simulink model "modelo_f_nico_local"  (R2024b)
settings: Solver=VariableStepAuto  StartTime=0.0  StopTime=100  RelTol=1e-3
InitFcn:
  | parametros
  | gain_CL
values from neighbouring files (symbols this model uses):
  Ah = [0 1 ... (first row only)    [calculo_observador_izaje.m]
  At = [ 0, 1, 0, 0 ... (first row only)    [calculo_observador_carro.m]
  b_cy = 1e7    (= 10000000)    [parametros.m]
  b_ha = -(J_hEq + (r_hd/(2*i_h))*m_l) * w_des_h*(1 + n_h + n_h^2) + b_hEq    [gain_CL.m]
  b_hb = 1e8    (= 100000000)    [parametros.m]
  b_hd = 8    [parametros.m]
  b_hEb = 2.2e9    (= 2200000000)    [parametros.m]
  b_hm = 18    [parametros.m]
  b_t = 90    [parametros.m]
  b_ta = M_tEq*w_des_t*(1+n_t+n_t^2)-b_tEq    [gain_CL.m]
  b_tb = 5e6    (= 5000000)    [parametros.m]
  b_td = 1.8    [parametros.m]
  b_tm = 6    [parametros.m]
  b_tw = 3e3    (= 3000)    [parametros.m]
  b_wu = 150    [parametros.m]
  Bch = [0 ... (first row only)    [calculo_observador_izaje.m]
  Bct = [ 0, 0 ... (first row only)    [calculo_observador_carro.m]
  Bdh = [0 ... (first row only)    [calculo_observador_izaje.m]
  Bdt = [ 0 ... (first row only)    [calculo_observador_carro.m]
  Ch = [1 0]    [calculo_observador_izaje.m]
  Ct = [ 1, 0, 0, 0 ]    [calculo_observador_carro.m]
  g = 9.80665    [parametros.m]
  i_h = 22    [parametros.m]
  i_t = 30    [parametros.m]
  J_hd_hEb = 3800    [parametros.m]
  J_hm_hb = 30    [parametros.m]
  J_td = 1200    [parametros.m]
  J_tm_tb = 7    [parametros.m]
  K_cy = 1.8e9    (= 1800000000)    [parametros.m]
  k_hsa = -(J_hEq + (r_hd/(2*i_h))*m_l) * w_des_h^2*(n_h + n_h^2 + n_h^3)    [gain_CL.m]
  k_hsia = -(J_hEq + (r_hd/(2*i_h))*m_l) * n_h^3 * w_des_h^3    [gain_CL.m]
  k_tsa = M_tEq*w_des_t^2*n_t*(1+n_t+n_t^2)    [gain_CL.m]
  k_tsia = M_tEq*w_des_t^3*n_t^3    [gain_CL.m]
  K_tw = 4.8e5    (= 480000)    [parametros.m]
  k_wu = 2.36e8    (= 236000000)    [parametros.m]
  l_h0 = (Y_t0-y_l0)    (= 5)    [parametros.m]
  Lh = place(Ah', Ch', polos_h)'    [calculo_observador_izaje.m]
  Lt = place(At', Ct', polos_deseados)'    [calculo_observador_carro.m]
  m_l = M_s+M_cmax    (= 65000)    [parametros.m]
  M_t = 30000    [parametros.m]
  M_tEq = i_t/r_td*(J_tm_tb+J_td/i_t^2)+r_td/i_t*(M_t+m_l)    (= 2083.33333333)    [parametros.m]
  r_hd = 0.75    [parametros.m]
  r_td = 0.50    (= 0.5)    [parametros.m]
  T_hbMax = 5e4    (= 50000)    [parametros.m]
  T_hEbMax = 1.1e6    (= 1100000)    [parametros.m]
  T_hmMax = 2e4    (= 20000)    [parametros.m]
  T_s = min([T_hs,T_ts])    [parametros.m]
  T_tbMax = 5e3    (= 5000)    [parametros.m]
  T_tmMax = 4e3    (= 4000)    [parametros.m]
  tau_tm = 1e-3    (= 0.001)    [parametros.m]
  theta_hm0 = -l_h0*i_h*2/r_hd    (= -293.333333333)    [parametros.m]
  theta_tm0 = (x_t0)*i_t/r_td    (= -1200)    [parametros.m]
  v_lx0 = 0    [parametros.m]
  v_ly0 = 0    [parametros.m]
  v_t0 = 0    [parametros.m]
  w_hm0 = 0    [parametros.m]
  w_hm_rated = v_h_max_load*2*i_h/r_hd    (= 88)    [parametros.m]
  w_tm0 = (v_t0)*i_t/r_td    (= 0)    [parametros.m]
  x_l0 = x_t0    (= -20)    [parametros.m]
  x_t0 = -20    [parametros.m]
  y_l0 = 40    [parametros.m]
  Y_t0 = 45    [parametros.m]
libraries: simulink x1
settings Model: Creator=nsorr  LastModifiedBy=nsorr

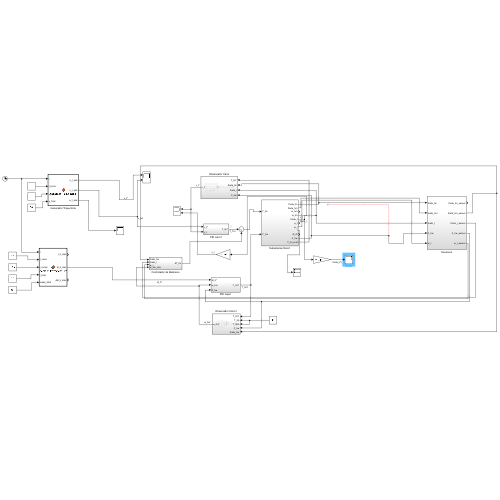
[thumbnail: Simulink's stored preview of the top-level diagram]
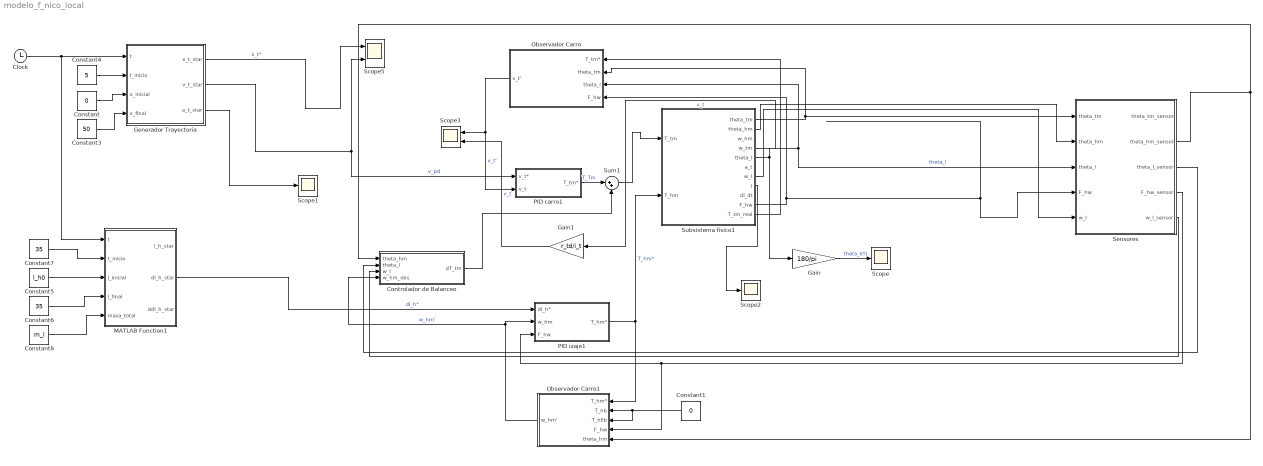
== system modelo_f_nico_local ==
  Clock : Clock
  Constant : Constant  Value=0
  Constant1 : Constant  Value=0
  Constant3 : Constant  Value=50
  Constant4 : Constant  Value=5
  Constant5 : Constant  Value=l_h0
  Constant6 : Constant  Value=35
  Constant7 : Constant  Value=35
  Constant8 : Constant  Value=m_l
  Controlador de Balanceo : Subsystem
  Gain : Gain  Gain=180/pi
  Gain1 : Gain  Gain=r_td/i_t
  Generador Trayectoria : MATLAB Function  TreatAsAtomicUnit=on
  MATLAB Function1 : MATLAB Function  TreatAsAtomicUnit=on
  Observador Carro : Subsystem
  Observador Carro1 : Subsystem
  PID carro1 : Subsystem
  PID izaje1 : Subsystem
  Scope : Scope
  Scope1 : Scope
  Scope2 : Scope
  Scope3 : Scope  NumInputPorts=2
  Scope5 : Scope  NumInputPorts=2
  Sensores : Subsystem
  Subsistema físico1 : Subsystem
  Sum1 : Sum  Inputs=|++
  wires:
  Generador Trayectoria/1(x_t_star) -> Scope5/1  "x_t*"
  MATLAB Function1/2(dl_h_star) -> PID izaje1/1(dl_h*)  "dl_h*"
  Subsistema físico1/2(theta_hm) -> Sensores/2(theta_hm)
  PID carro1/1(T_tm*) -> Sum1/1  "T_Tm"
  Subsistema físico1/8(l) -> Scope2/1
  Subsistema físico1/4(w_tm) -> Gain1/1  "v_t"
  Subsistema físico1/5(theta_l) -> Observador Carro/3(theta_l), Sensores/3(theta_l), Gain/1  "theta_l"
  PID izaje1/1(T_hm*) -> Observador Carro1/1(T_hm*), Subsistema físico1/2(T_hm)  "T_hm*"
  Gain/1 -> Scope/1  "theta_l(º)"
  Clock/1 -> MATLAB Function1/1(t), Generador Trayectoria/1(t)
  Constant/1 -> Generador Trayectoria/3(x_inicial)
  Constant3/1 -> Generador Trayectoria/4(x_final)
  Constant4/1 -> Generador Trayectoria/2(t_inicio)
  Constant5/1 -> MATLAB Function1/3(l_inicial)
  Constant6/1 -> MATLAB Function1/4(l_final)
  Constant7/1 -> MATLAB Function1/2(t_inicio)
  Constant8/1 -> MATLAB Function1/5(masa_total)
  Generador Trayectoria/2(v_t_star) -> PID carro1/1(v_t*), Scope5/2  "v_pd"
  Controlador de Balanceo/1(dT_tm) -> Sum1/2
  Sum1/1 -> Subsistema físico1/1(T_tm)
  Generador Trayectoria/3(a_t_star) -> Scope1/1
  Subsistema físico1/1(theta_tm) -> Observador Carro/2(theta_tm), Sensores/1(theta_tm)
  Subsistema físico1/10(F_hw) -> Observador Carro/4(F_hw), Sensores/4(F_hw)
  Subsistema físico1/7(w_l) -> Sensores/5(w_l)
  Sensores/5(w_l_sensor) -> Controlador de Balanceo/3(w_l)
  Sensores/3(theta_l_sensor) -> Controlador de Balanceo/2(theta_l)
  Sensores/2(theta_hm_sensor) -> Controlador de Balanceo/1(theta_hm), Observador Carro1/5(theta_hm)
  Sensores/4(F_hw_sensor) -> Observador Carro1/4(F_hw), PID izaje1/3(F_hw)
  Observador Carro1/1(w_hm') -> Controlador de Balanceo/4(w_hm_obs), PID izaje1/2(w_hm)  "w_hm'"
  Constant1/1 -> Observador Carro1/3(T_hEb), Observador Carro1/2(T_hb)
  Observador Carro/1(v_t') -> PID carro1/2(v_t), Scope3/1  "v_t'"
  Gain1/1 -> Scope3/2  "v_t"
  Subsistema físico1/11(T_tm_real) -> Observador Carro/1(T_tm*)

== system modelo_f_nico_local/Controlador de Balanceo ==
  theta_hm : Inport
  theta_l : Inport  Port=2
  w_l : Inport  Port=3
  w_hm_obs : Inport  Port=4
  Constant1 : Constant  Value=g
  Gain : Gain  Gain=r_hd/i_h/2
  Gain2 : Gain  Gain=M_tEq * r_td / i_t
  Gain3 : Gain  Gain=r_hd/i_h/2
  MATLAB Function : MATLAB Function  TreatAsAtomicUnit=on
  dT_tm : Outport
  wires:
  Gain3/1 -> MATLAB Function/3(l)
  theta_l/1 -> MATLAB Function/1(theta_l)
  Constant1/1 -> MATLAB Function/5(g)
  MATLAB Function/1(a_PD) -> Gain2/1
  theta_hm/1 -> Gain3/1
  Gain2/1 -> dT_tm/1
  w_l/1 -> MATLAB Function/2(w_l)
  w_hm_obs/1 -> Gain/1
  Gain/1 -> MATLAB Function/4(dl_dt)

== system modelo_f_nico_local/Observador Carro ==
  T_tm* : Inport
  theta_tm : Inport  Port=2
  theta_l : Inport  Port=3
  F_hw : Inport  Port=4
  Constant9 : Constant  Value=0
  Gain : Gain  Gain=r_td/i_t
  Mux : Mux
  Product : Product
  Sin : Trigonometry
  State-Space : StateSpace  A=At- Lt*Ct  B=[Bct, Bdt Lt]  C=[0, 1, 0, 0]  D=[0, 0, 0, 0]  InitialCondition=[0, 0, 0, 0]
  v_t' : Outport
  wires:
  Sin/1 -> Product/2
  Product/1 -> Mux/3
  Constant9/1 -> Mux/2
  theta_tm/1 -> Mux/4
  T_tm*/1 -> Mux/1
  Mux/1 -> State-Space/1
  theta_l/1 -> Sin/1
  F_hw/1 -> Product/1
  State-Space/1 -> Gain/1  "w_tm_obs'"
  Gain/1 -> v_t'/1

== system modelo_f_nico_local/Observador Carro1 ==
  T_hm* : Inport
  T_hb : Inport  Port=2
  T_hEb : Inport  Port=3
  F_hw : Inport  Port=4
  theta_hm : Inport  Port=5
  Mux : Mux  Inputs=5
  State-Space : StateSpace  A=Ah - Lh*Ch  B=[Bch, Bdh, Lh]  C=[0, 1]  D=[0, 0, 0, 0, 0]  InitialCondition=[theta_hm0, w_hm0]
  w_hm' : Outport
  wires:
  T_hb/1 -> Mux/2
  T_hm*/1 -> Mux/1
  Mux/1 -> State-Space/1
  T_hEb/1 -> Mux/3
  State-Space/1 -> w_hm'/1  "v_t'"
  F_hw/1 -> Mux/4
  theta_hm/1 -> Mux/5

== system modelo_f_nico_local/PID carro1 ==
  v_t* : Inport
  v_t : Inport  Port=2
  Gain : Gain  Gain=b_ta
  Gain1 : Gain  Gain=k_tsia
  Gain2 : Gain  Gain=k_tsa
  Integrator : Integrator  LimitOutput=on  UpperSaturationLimit=4e3  LowerSaturationLimit=-4e3
  Integrator1 : Integrator  LimitOutput=on  UpperSaturationLimit=4e3  LowerSaturationLimit=-4e3
  Sum : Sum  Inputs=|+-
  Sum1 : Sum  Inputs=+++
  T_tm* : Outport
  wires:
  Gain2/1 -> Sum1/2  "P"
  v_t*/1 -> Sum/1
  Gain/1 -> Sum1/3  "D"
  Gain1/1 -> Sum1/1  "I"
  Sum1/1 -> T_tm*/1
  Sum/1 -> Integrator1/1, Gain/1  "e"
  Integrator1/1 -> Integrator/1, Gain2/1
  Integrator/1 -> Gain1/1
  v_t/1 -> Sum/2  "v_t"

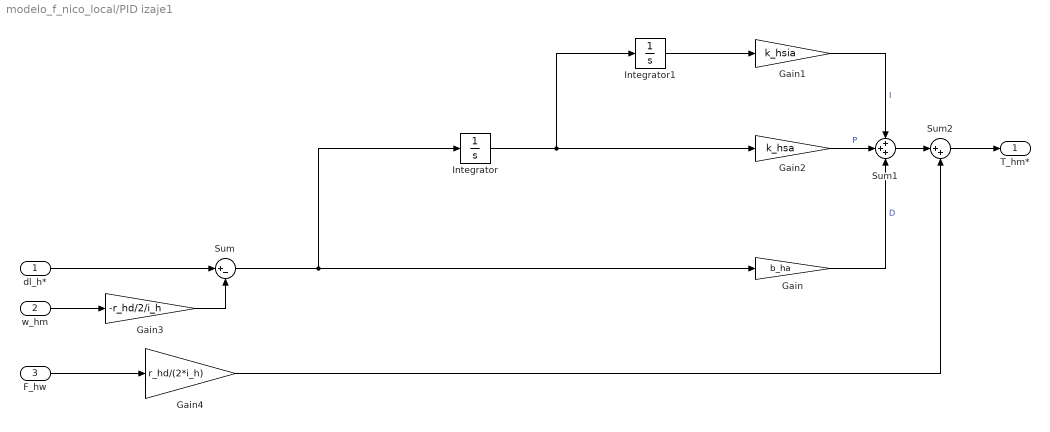
== system modelo_f_nico_local/PID izaje1 ==
  dl_h* : Inport
  w_hm : Inport  Port=2
  F_hw : Inport  Port=3
  Gain : Gain  Gain=b_ha
  Gain1 : Gain  Gain=k_hsia
  Gain2 : Gain  Gain=k_hsa
  Gain3 : Gain  Gain=-r_hd/2/i_h
  Gain4 : Gain  Gain=r_hd/(2*i_h)
  Integrator : Integrator
  Integrator1 : Integrator
  Sum : Sum  Inputs=|+-
  Sum1 : Sum  Inputs=+++
  Sum2 : Sum  Inputs=|++
  T_hm* : Outport
  wires:
  Gain2/1 -> Sum1/2  "P"
  dl_h*/1 -> Sum/1
  Gain/1 -> Sum1/3  "D"
  Gain1/1 -> Sum1/1  "I"
  w_hm/1 -> Gain3/1
  Sum1/1 -> Sum2/1
  Sum/1 -> Integrator/1, Gain/1
  Integrator/1 -> Integrator1/1, Gain2/1
  Integrator1/1 -> Gain1/1
  Gain3/1 -> Sum/2
  Sum2/1 -> T_hm*/1
  Gain4/1 -> Sum2/2
  F_hw/1 -> Gain4/1

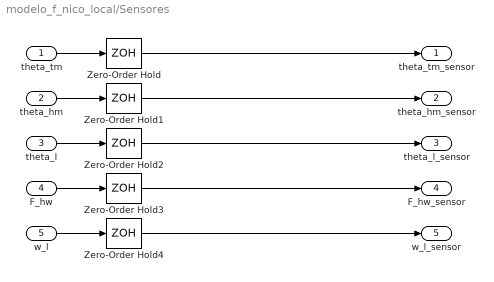
== system modelo_f_nico_local/Sensores ==
  theta_tm : Inport
  theta_hm : Inport  Port=2
  theta_l : Inport  Port=3
  F_hw : Inport  Port=4
  w_l : Inport  Port=5
  Zero-Order Hold{,1..4} (5 alike) : ZeroOrderHold  SampleTime=T_s
  theta_tm_sensor : Outport
  theta_hm_sensor : Outport  Port=2
  theta_l_sensor : Outport  Port=3
  F_hw_sensor : Outport  Port=4
  w_l_sensor : Outport  Port=5
  wires:
  theta_tm/1 -> Zero-Order Hold/1
  Zero-Order Hold/1 -> theta_tm_sensor/1
  Zero-Order Hold1/1 -> theta_hm_sensor/1
  theta_hm/1 -> Zero-Order Hold1/1
  w_l/1 -> Zero-Order Hold4/1
  F_hw/1 -> Zero-Order Hold3/1
  theta_l/1 -> Zero-Order Hold2/1
  Zero-Order Hold2/1 -> theta_l_sensor/1
  Zero-Order Hold3/1 -> F_hw_sensor/1
  Zero-Order Hold4/1 -> w_l_sensor/1

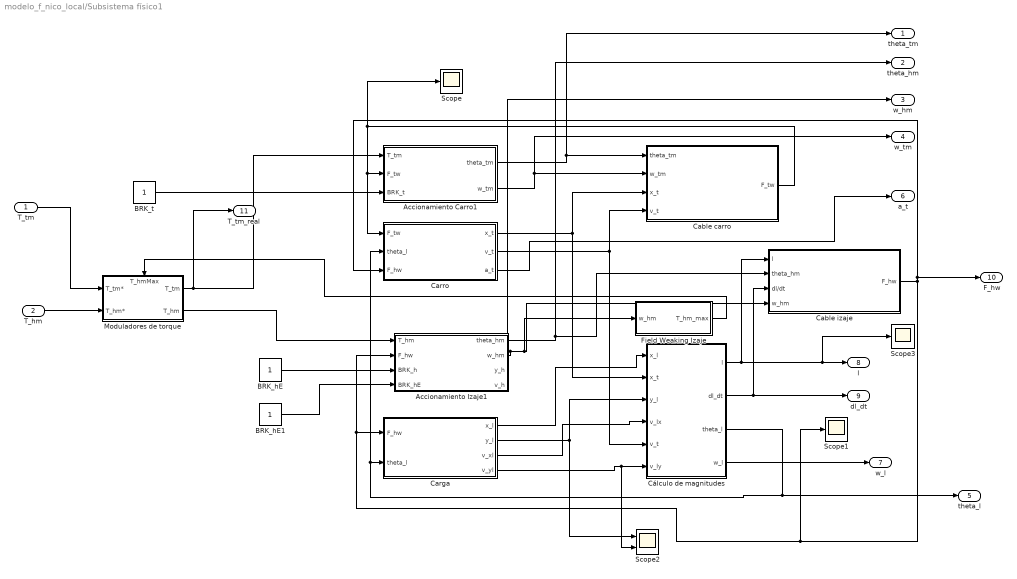
== system modelo_f_nico_local/Subsistema físico1 ==
  T_tm : Inport
  T_hm : Inport  Port=2
  Accionamiento Carro1 : Subsystem
  Accionamiento Izaje1 : Subsystem
  BRK_hE : Constant
  BRK_hE1 : Constant
  BRK_t : Constant
  Cable carro : Subsystem
  Cable izaje : Subsystem
  Carga : Subsystem
  Carro : Subsystem
  Cálculo de magnitudes : Subsystem
  Field Weaking Izaje : Subsystem
  Moduladores de torque : Subsystem
      settings: PortSchema="{\"entries\":[{\"content\":{\"sides\":[{\"content\":{\"connectorIds\":[\"In1\",\"In2\"]},\"type\":\"ConnectorPlacement.EquallySpacedRectSide\",\"uuid\":\"c66d3892-523c-433a-8dde-517eb495bac1\"},{\"content\":{\"connectorIds\":[\"Out1\",\"Out2\"],\"side\":\"RIGHT\"},\"type\":\"ConnectorPlacement.EquallySpacedRectSide\",\"uuid\":\"bbb0a9b0-6ff9-4fa8-ace8-11da5b7abadd\"},{\"content\":{\"connectorIds\":[\"In3\"],\"side\":\"TOP\"},\"type\":\"ConnectorPlacement.EquallySpacedRectSide\",\"uuid\":\"35baaaad-8e6c-401a-84f7-749de5492b29\"}]},\"type\":\"ConnectorPlacement.EquallySpacedConnector\",\"uuid\":\"d8d05b6c-004b-40f1-854a-ea077232777a\"}],\"packageUris\":[\"http://schema.mathworks.com/mf0/Connector/R2020b\"],\"version\":\"1.0\"}"
  Scope : Scope
  Scope1 : Scope
  Scope2 : Scope  NumInputPorts=2
  Scope3 : Scope
  theta_tm : Outport
  theta_hm : Outport  Port=2
  w_hm : Outport  Port=3
  w_tm : Outport  Port=4
  theta_l : Outport  Port=5
  a_t : Outport  Port=6
  w_l : Outport  Port=7
  l : Outport  Port=8
  dl_dt : Outport  Port=9
  F_hw : Outport  Port=10
  T_tm_real : Outport  Port=11
  wires:
  Accionamiento Carro1/1(theta_tm) -> theta_tm/1, Cable carro/1(theta_tm)
  Accionamiento Carro1/2(w_tm) -> w_tm/1, Cable carro/2(w_tm)
  Carro/1(x_t) -> Cálculo de magnitudes/2(x_t), Cable carro/3(x_t)
  Carro/2(v_t) -> Cálculo de magnitudes/5(v_t), Cable carro/4(v_t)
  Cable carro/1(F_tw) -> Scope/1, Carro/1(F_tw), Accionamiento Carro1/2(F_tw)
  Carga/1(x_l) -> Cálculo de magnitudes/1(x_l)
  Carga/2(y_l) -> Cálculo de magnitudes/3(y_l), Scope2/1
  Carga/3(v_xl) -> Cálculo de magnitudes/4(v_lx)
  Carga/4(v_yl) -> Cálculo de magnitudes/6(v_ly), Scope2/2
  Cálculo de magnitudes/1(l) -> Cable izaje/1(l), Scope3/1, l/1
  Accionamiento Izaje1/1(theta_hm) -> theta_hm/1, Cable izaje/2(theta_hm)
  Accionamiento Izaje1/2(w_hm) -> w_hm/1, Field Weaking Izaje/1(w_hm), Cable izaje/4(w_hm)
  Cable izaje/1(F_hw) -> F_hw/1, Carro/3(F_hw), Accionamiento Izaje1/2(F_hw), Carga/1(F_hw), Scope1/1
  Cálculo de magnitudes/2(dl_dt) -> Cable izaje/3(dl/dt), dl_dt/1
  Carro/3(a_t) -> a_t/1
  Cálculo de magnitudes/3(theta_l) -> Carro/2(theta_l), Carga/2(theta_l), theta_l/1
  Cálculo de magnitudes/4(w_l) -> w_l/1
  BRK_t/1 -> Accionamiento Carro1/3(BRK_t)
  BRK_hE/1 -> Accionamiento Izaje1/3(BRK_h)
  BRK_hE1/1 -> Accionamiento Izaje1/4(BRK_hE)
  T_tm/1 -> Moduladores de torque/1(T_tm*)
  T_hm/1 -> Moduladores de torque/2(T_hm*)
  Field Weaking Izaje/1(T_hm_max) -> Moduladores de torque/3(T_hmMax)
  Moduladores de torque/2(T_hm) -> Accionamiento Izaje1/1(T_hm)
  Moduladores de torque/1(T_tm) -> T_tm_real/1, Accionamiento Carro1/1(T_tm)

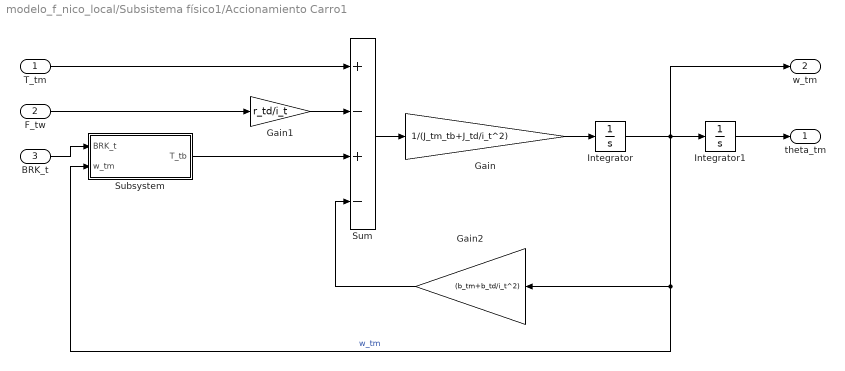
== system modelo_f_nico_local/Subsistema físico1/Accionamiento Carro1 ==
  T_tm : Inport
  F_tw : Inport  Port=2
  BRK_t : Inport  Port=3
  Gain : Gain  Gain=1/(J_tm_tb+J_td/i_t^2)
  Gain1 : Gain  Gain=r_td/i_t
  Gain2 : Gain  Gain=(b_tm+b_td/i_t^2)
  Integrator : Integrator  InitialCondition=w_tm0
  Integrator1 : Integrator  InitialCondition=theta_tm0
  Subsystem : Subsystem
  Sum : Sum  Inputs=+-+-
  theta_tm : Outport
  w_tm : Outport  Port=2
  wires:
  Integrator1/1 -> theta_tm/1
  Integrator/1 -> w_tm/1, Gain2/1, Subsystem/2(w_tm), Integrator1/1  "w_tm"
  Gain/1 -> Integrator/1
  Sum/1 -> Gain/1
  T_tm/1 -> Sum/1
  F_tw/1 -> Gain1/1
  Gain1/1 -> Sum/2
  Subsystem/1(T_tb) -> Sum/3
  Gain2/1 -> Sum/4
  BRK_t/1 -> Subsystem/1(BRK_t)

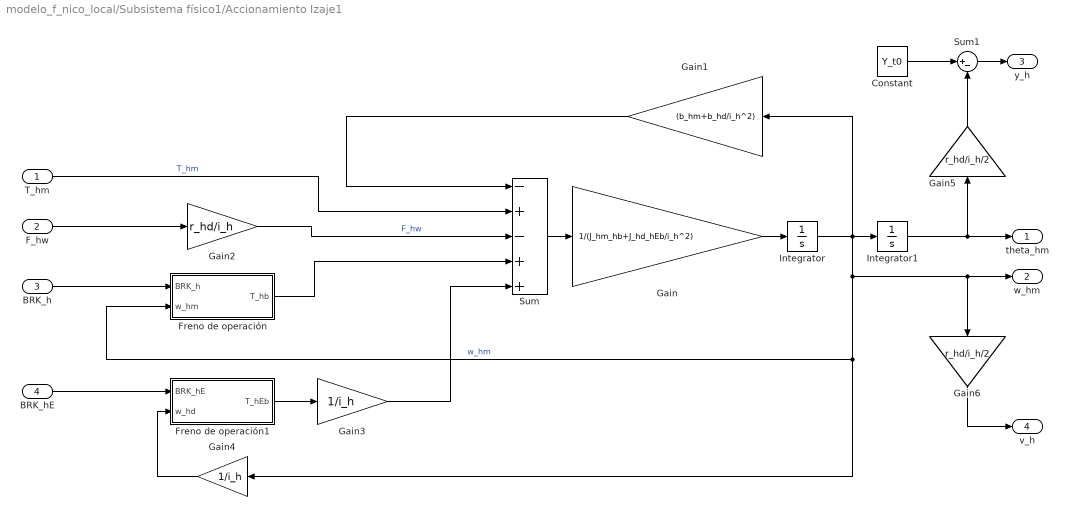
== system modelo_f_nico_local/Subsistema físico1/Accionamiento Izaje1 ==
  T_hm : Inport
  F_hw : Inport  Port=2
  BRK_h : Inport  Port=3
  BRK_hE : Inport  Port=4
  Constant : Constant  Value=Y_t0
  Freno de operación : Subsystem
  Freno de operación1 : Subsystem
  Gain : Gain  Gain=1/(J_hm_hb+J_hd_hEb/i_h^2)
  Gain1 : Gain  Gain=(b_hm+b_hd/i_h^2)
  Gain2 : Gain  Gain=r_hd/i_h
  Gain3 : Gain  Gain=1/i_h
  Gain4 : Gain  Gain=1/i_h
  Gain5 : Gain  Gain=r_hd/i_h/2
  Gain6 : Gain  Gain=r_hd/i_h/2
  Integrator : Integrator  InitialCondition=w_hm0
  Integrator1 : Integrator  InitialCondition=theta_hm0
  Sum : Sum  Inputs=-+-++
  Sum1 : Sum  Inputs=|+-
  theta_hm : Outport
  w_hm : Outport  Port=2
  y_h : Outport  Port=3
  v_h : Outport  Port=4
  wires:
  Integrator1/1 -> Gain5/1, theta_hm/1
  Integrator/1 -> Integrator1/1, Gain6/1, w_hm/1, Gain4/1, Freno de operación/2(w_hm), Gain1/1  "w_hm"
  Gain/1 -> Integrator/1
  Sum/1 -> Gain/1
  Gain1/1 -> Sum/1
  F_hw/1 -> Gain2/1
  Gain2/1 -> Sum/3  "F_hw"
  T_hm/1 -> Sum/2  "T_hm"
  Freno de operación/1(T_hb) -> Sum/4
  BRK_h/1 -> Freno de operación/1(BRK_h)
  Freno de operación1/1(T_hEb) -> Gain3/1
  Gain3/1 -> Sum/5
  BRK_hE/1 -> Freno de operación1/1(BRK_hE)
  Gain4/1 -> Freno de operación1/2(w_hd)
  Sum1/1 -> y_h/1
  Gain5/1 -> Sum1/2
  Constant/1 -> Sum1/1
  Gain6/1 -> v_h/1

== system modelo_f_nico_local/Subsistema físico1/Cable carro ==
  theta_tm : Inport
  w_tm : Inport  Port=2
  x_t : Inport  Port=3
  v_t : Inport  Port=4
  Gain : Gain  Gain=b_tw
  Gain1 : Gain  Gain=K_tw
  Gain2 : Gain  Gain=r_td/i_t
  Gain3 : Gain  Gain=r_td/i_t
  Sum : Sum  Inputs=|+-
  Sum1 : Sum  Inputs=|+-
  Sum2 : Sum  Inputs=|++
  F_tw : Outport
  wires:
  Sum/1 -> Gain1/1
  theta_tm/1 -> Gain3/1
  x_t/1 -> Sum/2
  Sum1/1 -> Gain/1
  w_tm/1 -> Gain2/1
  v_t/1 -> Sum1/2
  Gain/1 -> Sum2/2
  Gain1/1 -> Sum2/1
  Sum2/1 -> F_tw/1
  Gain2/1 -> Sum1/1  "v_td"
  Gain3/1 -> Sum/1  "x_td"

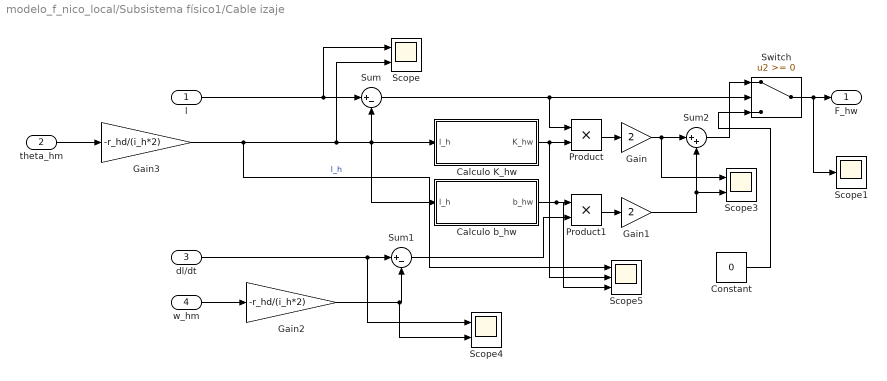
== system modelo_f_nico_local/Subsistema físico1/Cable izaje ==
  l : Inport
  theta_hm : Inport  Port=2
  dl/dt : Inport  Port=3
  w_hm : Inport  Port=4
  Calculo K_hw : Subsystem
  Calculo b_hw : Subsystem
  Constant : Constant  Value=0
  Gain : Gain  Gain=2
  Gain1 : Gain  Gain=2
  Gain2 : Gain  Gain=-r_hd/(i_h*2)
  Gain3 : Gain  Gain=-r_hd/(i_h*2)
  Product : Product
  Product1 : Product
  Scope : Scope  NumInputPorts=2
  Scope1 : Scope
  Scope3 : Scope  NumInputPorts=2
  Scope4 : Scope  NumInputPorts=2
  Scope5 : Scope  NumInputPorts=3
  Sum : Sum  Inputs=|+-
  Sum1 : Sum  Inputs=|+-
  Sum2 : Sum  Inputs=|++
  Switch : Switch  SaturateOnIntegerOverflow=off  InputSameDT=off
  F_hw : Outport
  wires:
  l/1 -> Scope/1, Sum/1
  theta_hm/1 -> Gain3/1
  Sum/1 -> Product/1, Switch/2
  Calculo K_hw/1(K_hw) -> Scope5/2, Product/2
  Product/1 -> Gain/1
  w_hm/1 -> Gain2/1
  Product1/1 -> Gain1/1
  Calculo b_hw/1(b_hw) -> Scope5/3, Product1/1
  Gain1/1 -> Scope3/2, Sum2/2
  Gain/1 -> Scope3/1, Sum2/1
  Sum2/1 -> Switch/1
  Switch/1 -> Scope1/1, F_hw/1
  dl/dt/1 -> Scope4/1, Sum1/1
  Constant/1 -> Switch/3
  Gain2/1 -> Scope4/2, Sum1/2
  Gain3/1 -> Scope5/1, Calculo b_hw/1(l_h), Calculo K_hw/1(l_h), Sum/2, Scope/2  "l_h"
  Sum1/1 -> Product1/2

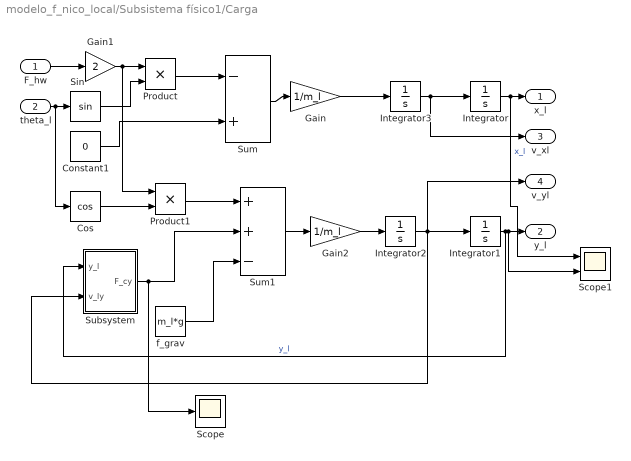
== system modelo_f_nico_local/Subsistema físico1/Carga ==
  F_hw : Inport
  theta_l : Inport  Port=2
  Constant1 : Constant  Value=0
  Cos : Trigonometry  Operator=cos
  Gain : Gain  Gain=1/m_l
  Gain1 : Gain  Gain=2
  Gain2 : Gain  Gain=1/m_l
  Integrator : Integrator  InitialCondition=x_l0
  Integrator1 : Integrator  InitialCondition=y_l0
  Integrator2 : Integrator  InitialCondition=v_ly0
  Integrator3 : Integrator  InitialCondition=v_lx0
  Product : Product
  Product1 : Product
  Scope : Scope
  Scope1 : Scope  NumInputPorts=2
  Sin : Trigonometry
  Subsystem : Subsystem
  Sum : Sum  Inputs=-+
  Sum1 : Sum  Inputs=++-
  f_grav : Constant  Value=m_l*g
  x_l : Outport
  y_l : Outport  Port=2
  v_xl : Outport  Port=3
  v_yl : Outport  Port=4
  wires:
  Sum/1 -> Gain/1
  Gain/1 -> Integrator3/1
  theta_l/1 -> Cos/1, Sin/1
  F_hw/1 -> Gain1/1
  Gain1/1 -> Product/1, Product1/1
  Sin/1 -> Product/2
  Product/1 -> Sum/1
  Constant1/1 -> Sum/2
  Product1/1 -> Sum1/1
  Cos/1 -> Product1/2
  f_grav/1 -> Sum1/3
  Subsystem/1(F_cy) -> Scope/1, Sum1/2
  Gain2/1 -> Integrator2/1
  Sum1/1 -> Gain2/1
  Integrator/1 -> Scope1/1, x_l/1  "x_l"
  Integrator3/1 -> v_xl/1, Integrator/1
  Integrator2/1 -> v_yl/1, Subsystem/2(v_ly), Integrator1/1
  Integrator1/1 -> Subsystem/1(y_l), Scope1/2, y_l/1  "y_l"

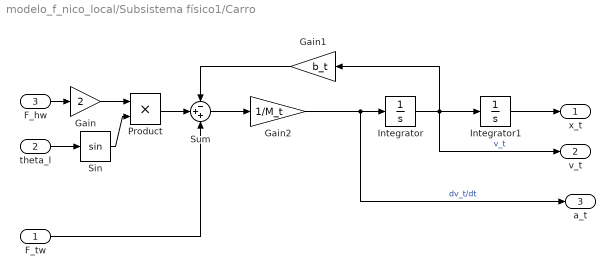
== system modelo_f_nico_local/Subsistema físico1/Carro ==
  F_tw : Inport
  theta_l : Inport  Port=2
  F_hw : Inport  Port=3
  Gain : Gain  Gain=2
  Gain1 : Gain  Gain=b_t
  Gain2 : Gain  Gain=1/M_t
  Integrator : Integrator  InitialCondition=v_t0
  Integrator1 : Integrator  InitialCondition=x_t0
  Product : Product
  Sin : Trigonometry
  Sum : Sum  Inputs=-++
  x_t : Outport
  v_t : Outport  Port=2
  a_t : Outport  Port=3
  wires:
  F_tw/1 -> Sum/3
  F_hw/1 -> Gain/1
  Gain/1 -> Product/1
  theta_l/1 -> Sin/1
  Sin/1 -> Product/2
  Product/1 -> Sum/2
  Integrator/1 -> v_t/1, Integrator1/1, Gain1/1  "v_t"
  Sum/1 -> Gain2/1
  Gain2/1 -> a_t/1, Integrator/1  "dv_t/dt"
  Integrator1/1 -> x_t/1
  Gain1/1 -> Sum/1

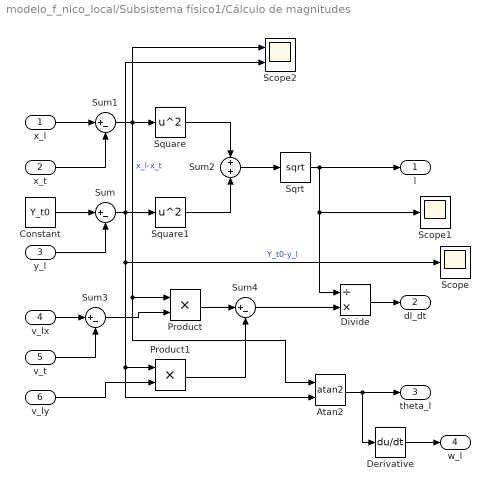
== system modelo_f_nico_local/Subsistema físico1/Cálculo de magnitudes ==
  x_l : Inport
  x_t : Inport  Port=2
  y_l : Inport  Port=3
  v_lx : Inport  Port=4
  v_t : Inport  Port=5
  v_ly : Inport  Port=6
  Atan2 : Trigonometry  Operator=atan2
  Constant : Constant  Value=Y_t0
  Derivative : Derivative
  Divide : Product  Inputs=/*
  Product : Product
  Product1 : Product
  Scope : Scope
  Scope1 : Scope
  Scope2 : Scope  NumInputPorts=2
  Sqrt : Sqrt
  Square : Math  Operator=square
  Square1 : Math  Operator=square
  Sum{,1,3..4} (4 alike) : Sum  Inputs=|+-
  Sum2 : Sum  Inputs=+|+
  l : Outport
  dl_dt : Outport  Port=2
  theta_l : Outport  Port=3
  w_l : Outport  Port=4
  wires:
  Constant/1 -> Sum/1
  y_l/1 -> Sum/2
  x_l/1 -> Sum1/1
  x_t/1 -> Sum1/2
  Sum1/1 -> Scope2/1, Atan2/1, Product/1, Square/1  "x_l-x_t"
  Sum/1 -> Scope2/2, Atan2/2, Product1/1, Scope/1, Square1/1  "Y_t0-y_l"
  Square/1 -> Sum2/1
  Square1/1 -> Sum2/2
  Sum2/1 -> Sqrt/1
  Sqrt/1 -> Divide/1, Scope1/1, l/1
  v_lx/1 -> Sum3/1
  v_t/1 -> Sum3/2
  Sum3/1 -> Product/2
  Product/1 -> Sum4/1
  v_ly/1 -> Product1/2
  Product1/1 -> Sum4/2
  Sum4/1 -> Divide/2
  Divide/1 -> dl_dt/1
  Atan2/1 -> Derivative/1, theta_l/1
  Derivative/1 -> w_l/1

== system modelo_f_nico_local/Subsistema físico1/Field Weaking Izaje ==
  w_hm : Inport
  Abs : Abs  SaturateOnIntegerOverflow=off
  Constant : Constant  Value=w_hm_rated
  Divide : Product  Inputs=*/
  Gain : Gain  Gain=T_hmMax
  Max : MinMax  Function=max  Inputs=2
  Square : Math  Operator=square
  T_hm_max : Outport
  wires:
  w_hm/1 -> Abs/1
  Constant/1 -> Divide/1, Max/2
  Divide/1 -> Square/1
  Square/1 -> Gain/1
  Gain/1 -> T_hm_max/1
  Abs/1 -> Max/1
  Max/1 -> Divide/2

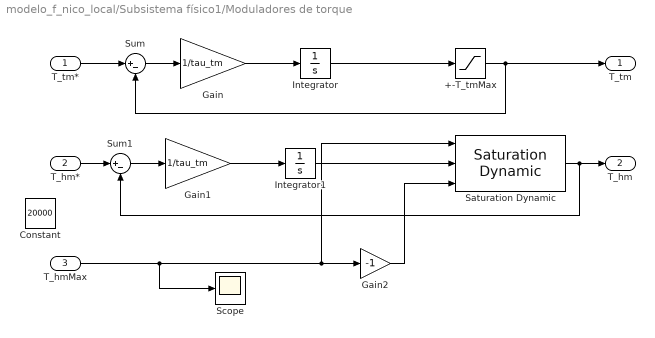
== system modelo_f_nico_local/Subsistema físico1/Moduladores de torque ==
  T_tm* : Inport
  T_hm* : Inport  Port=2
  T_hmMax : Inport  Port=3
  +-T_tmMax : Saturate  UpperLimit=+T_tmMax  LowerLimit=-T_tmMax
  Constant : Constant  Value=20000
  Gain : Gain  Gain=1/tau_tm
  Gain1 : Gain  Gain=1/tau_tm
  Gain2 : Gain  Gain=-1
  Integrator : Integrator
  Integrator1 : Integrator
  Saturation Dynamic : simulink/Discontinuities/Saturation Dynamic  OutMin=[]  OutMax=[]  OutDataTypeStr=Inherit: Same as second input  OutDataType=fixdt(1, 16)  OutScaling=2^-10  DoSatur=off
  Scope : Scope
  Sum : Sum  Inputs=|+-
  Sum1 : Sum  Inputs=|+-
  T_tm : Outport
  T_hm : Outport  Port=2
  wires:
  +-T_tmMax/1 -> Sum/2, T_tm/1
  Gain/1 -> Integrator/1
  Integrator/1 -> +-T_tmMax/1
  T_tm*/1 -> Sum/1
  Sum/1 -> Gain/1
  Gain1/1 -> Integrator1/1
  Sum1/1 -> Gain1/1
  Integrator1/1 -> Saturation Dynamic/2
  T_hm*/1 -> Sum1/1
  Saturation Dynamic/1 -> Sum1/2, T_hm/1
  Gain2/1 -> Saturation Dynamic/3
  T_hmMax/1 -> Scope/1, Saturation Dynamic/1, Gain2/1

== system modelo_f_nico_local/Subsistema físico1/Accionamiento Carro1/Subsystem ==
  BRK_t : Inport
  w_tm : Inport  Port=2
  +-T_tbmax : Saturate  UpperLimit=T_tbMax  LowerLimit=-T_tbMax
  Constant : Constant  Value=0
  Gain : Gain  Gain=-b_tb
  Gain1 : Gain  Gain=-T_tbMax
  Switch : Switch  Criteria=u2 > Threshold  SaturateOnIntegerOverflow=off  InputSameDT=off
  Tanh : Trigonometry  Operator=tanh
  T_tb : Outport
  wires:
  BRK_t/1 -> Switch/2
  Constant/1 -> Switch/1
  Gain/1 -> Tanh/1
  w_tm/1 -> Gain/1
  Switch/1 -> +-T_tbmax/1
  +-T_tbmax/1 -> T_tb/1
  Tanh/1 -> Gain1/1
  Gain1/1 -> Switch/3

== system modelo_f_nico_local/Subsistema físico1/Accionamiento Izaje1/Freno de operación ==
  BRK_h : Inport
  w_hm : Inport  Port=2
  +-T_hbmax : Saturate  UpperLimit=T_hbMax  LowerLimit=-T_hbMax
  Constant : Constant  Value=0
  Gain : Gain  Gain=b_hb
  Gain1 : Gain  Gain=-T_hbMax
  Switch : Switch  Criteria=u2 > Threshold  SaturateOnIntegerOverflow=off  InputSameDT=off
  Tanh : Trigonometry  Operator=tanh
  T_hb : Outport
  wires:
  BRK_h/1 -> Switch/2
  Constant/1 -> Switch/1
  Gain/1 -> Tanh/1
  w_hm/1 -> Gain/1
  Switch/1 -> +-T_hbmax/1
  +-T_hbmax/1 -> T_hb/1
  Tanh/1 -> Gain1/1
  Gain1/1 -> Switch/3

== system modelo_f_nico_local/Subsistema físico1/Accionamiento Izaje1/Freno de operación1 ==
  BRK_hE : Inport
  w_hd : Inport  Port=2
  +-T_hEbmax : Saturate  UpperLimit=T_hEbMax  LowerLimit=-T_hEbMax
  Constant : Constant  Value=0
  Gain : Gain  Gain=b_hEb
  Gain1 : Gain  Gain=-T_hEbMax
  Switch : Switch  Criteria=u2 > Threshold  SaturateOnIntegerOverflow=off  InputSameDT=off
  Tanh : Trigonometry  Operator=tanh
  T_hEb : Outport
  wires:
  BRK_hE/1 -> Switch/2
  Constant/1 -> Switch/1
  Gain/1 -> Tanh/1
  w_hd/1 -> Gain/1
  Switch/1 -> +-T_hEbmax/1
  +-T_hEbmax/1 -> T_hEb/1
  Tanh/1 -> Gain1/1
  Gain1/1 -> Switch/3

== system modelo_f_nico_local/Subsistema físico1/Cable izaje/Calculo K_hw ==
  l_h : Inport
  Constant : Constant  Value=110
  Constant1 : Constant  Value=k_wu
  Divide : Product  Inputs=*/
  Gain : Gain  Gain=2
  Sum : Sum  Inputs=|++
  K_hw : Outport
  wires:
  l_h/1 -> Gain/1
  Gain/1 -> Sum/1
  Constant/1 -> Sum/2
  Sum/1 -> Divide/2
  Constant1/1 -> Divide/1
  Divide/1 -> K_hw/1

== system modelo_f_nico_local/Subsistema físico1/Cable izaje/Calculo b_hw ==
  l_h : Inport
  Constant : Constant  Value=110
  Gain : Gain  Gain=2
  Gain1 : Gain  Gain=b_wu
  Sum : Sum  Inputs=|++
  b_hw : Outport
  wires:
  l_h/1 -> Gain/1
  Gain/1 -> Sum/1
  Constant/1 -> Sum/2
  Sum/1 -> Gain1/1
  Gain1/1 -> b_hw/1

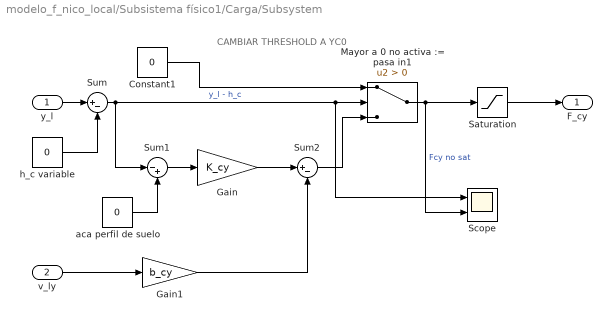
== system modelo_f_nico_local/Subsistema físico1/Carga/Subsystem ==
  note: CAMBIAR THRESHOLD A YC0
  y_l : Inport
  v_ly : Inport  Port=2
  Constant1 : Constant  Value=0
  Gain : Gain  Gain=K_cy
  Gain1 : Gain  Gain=b_cy
  Mayor a 0 no activa := pasa in1 : Switch  Criteria=u2 > Threshold  SaturateOnIntegerOverflow=off  InputSameDT=off
  Saturation : Saturate  UpperLimit=inf  LowerLimit=0
  Scope : Scope  NumInputPorts=2
  Sum : Sum  Inputs=|+-
  Sum1 : Sum  Inputs=|-+
  Sum2 : Sum  Inputs=|+-
  aca perfil de suelo : Constant  Value=0
  h_c variable : Constant  Value=0
  F_cy : Outport
  wires:
  Mayor a 0 no activa := pasa in1/1 -> Scope/2, Saturation/1  "Fcy no sat"
  Sum2/1 -> Mayor a 0 no activa := pasa in1/3
  Constant1/1 -> Mayor a 0 no activa := pasa in1/1
  Sum/1 -> Sum1/1, Scope/1, Mayor a 0 no activa := pasa in1/2  "y_l - h_c"
  y_l/1 -> Sum/1
  h_c variable/1 -> Sum/2
  aca perfil de suelo/1 -> Sum1/2
  Sum1/1 -> Gain/1
  Gain/1 -> Sum2/1
  v_ly/1 -> Gain1/1
  Gain1/1 -> Sum2/2
  Saturation/1 -> F_cy/1

== matlab function modelo_f_nico_local/Generador Trayectoria ==
  data: t input; t_inicio input; x_t_star output; x_inicial input; x_final input; v_t_star output; a_t_star output
function [x_t_star, v_t_star, a_t_star] = generador_trayectoria(t, t_inicio, x_inicial, x_final)
    % ---------------------------------------------------------------------
    % LIMITES OPERATIVOS (Sección 3.3) - PERFIL EN "S" (Jerk Limitado)
    % ---------------------------------------------------------------------
    v_max_limite = 4.0; % [m/s]
    a_max_limite = 0.8; % [m/s^2]
    
    % ESCUDO DE ESPERA
    if t < t_inicio
        x_t_star = x_inicial;
        v_t_star = 0;
        a_t_star = 0;
        return;
    end
    
    t_eff = t - t_inicio;
    D = abs(x_final - x_inicial);
    dir = sign(x_final - x_inicial);
    
    if D == 0
        x_t_star = x_inicial;
        v_t_star = 0;
        a_t_star = 0;
        return;
    end
    
    % ---------------------------------------------------------------------
    % CALCULO DEL PERFIL SENOIDAL (S-Curve)
    % ---------------------------------------------------------------------
    % Tiempo y distancia teórica para aceleración senoidal completa
    t_a = (pi * v_max_limite) / (2 * a_max_limite);
    d_a = (v_max_limite * t_a) / 2;
    
    if 2 * d_a >= D
        % El trayecto es corto: No llega a velocidad crucero (Perfil campana)
        v_pico = sqrt((2 * a_max_limite * D) / pi);
        t_a = (pi * v_pico) / (2 * a_max_limite);
        t_crucero = 0;
        v_crucero = v_pico;
        d_crucero = 0;
        d_a = D / 2;
    else
        % El trayecto es largo: Perfil en "S" con tramo de crucero plano
        v_crucero = v_max_limite;
        d_crucero = D - 2 * d_a;
        t_crucero = d_crucero / v_crucero;
    end
    
    t_total = 2 * t_a + t_crucero;
    
    % ---------------------------------------------------------------------
    % ECUACIONES CINEMÁTICAS INTEGRADAS (Onda Seno)
    % ---------------------------------------------------------------------
    if t_eff < t_a
        % Fase 1: Aceleración Suave (Onda Seno)
        a_t_star = a_max_limite * sin(pi * t_eff / t_a) * dir;
        v_t_star = (a_max_limite * t_a / pi) * (1 - cos(pi * t_eff / t_a)) * dir;
        x_t_star = x_inicial + ((a_max_limite * t_a / pi) * (t_eff - (t_a / pi) * sin(pi * t_eff / t_a))) * dir;
        
    elseif t_eff < (t_a + t_crucero)
        % Fase 2: Velocidad Constante (Crucero)
        t_fase2 = t_eff - t_a;
        a_t_star = 0;
        v_t_star = v_crucero * dir;
        x_t_star = x_inicial + d_a * dir + v_crucero * t_fase2 * dir;
        
    elseif t_eff < t_total
        % Fase 3: Desaceleración Suave (Onda Seno invertida)
        t_fase3 = t_eff - (t_a + t_crucero);
        a_t_star = -a_max_limite * sin(pi * t_fase3 / t_a) * dir;
        v_t_star = (v_crucero - (a_max_limite * t_a / pi) * (1 - cos(pi * t_fase3 / t_a))) * dir;
        x_t_star = x_inicial + (d_a + d_crucero) * dir + (v_crucero * t_fase3 - (a_max_limite * t_a / pi) * (t_fase3 - (t_a / pi) * sin(pi * t_fase3 / t_a))) * dir;
        
    else
        % Fase 4: Destino
        x_t_star = x_final;
        v_t_star = 0;
        a_t_star = 0;
    end
end

== matlab function modelo_f_nico_local/Controlador de Balanceo/MATLAB Function ==
  data: theta_l input; a_PD output; w_l input; l input; dl_dt input; g input
function a_PD = controlador_balanceo(theta_l, w_l, l, dl_dt, g)
    % 1. Escudos de seguridad
    if l < 0.1
        l_seguro = 0.1;
    else
        l_seguro = l;
    end

    theta_max = 80 * (pi/180);
    if theta_l > theta_max
        theta_math = theta_max;
    elseif theta_l < -theta_max
        theta_math = -theta_max;
    else
        theta_math = theta_l;
    end

    if abs(theta_math) < 1e-4
        sinc_theta = 1;
    else
        sinc_theta = sin(theta_math) / theta_math;
    end

    % 2. EL CORTACORRIENTE (ZONA MUERTA)
    % Apaga nuestra corrección si el péndulo ya casi no se mueve
    if abs(theta_math) < 0.005 && abs(w_l) < 0.01
        a_PD = 0;
        return; 
    end

    % 3. Frecuencia natural dinámica (Opción 1)
    w_o = 2*sqrt(g / l_seguro);

    % 4. Fórmulas LPV
    K_po = (g * sinc_theta - (w_o^2) * l_seguro) / cos(theta_math);
    K_do = (2 * dl_dt - 2 * w_o * l_seguro) / cos(theta_math);

    % 5. Salida de control
    a_PD = - K_po * theta_l - K_do * w_l;
end

== matlab function modelo_f_nico_local/MATLAB Function1 ==
  data: t input; l_h_star output; t_inicio input; l_inicial input; l_final input; masa_total input; dl_h_star output; ddl_h_star output
function [l_h_star, dl_h_star, ddl_h_star] = generador_trayectoria_izaje(t, t_inicio, l_inicial, l_final, masa_total)
    % ---------------------------------------------------------------------
    % CONSTANTES FISICAS Y OPERATIVAS DE IZAJE (Sección 3.3 y 3.5)
    % ---------------------------------------------------------------------
    g = 9.80665;               % [m/s^2]
    P_const = 956150;          % [W] Potencia máxima (956.15 kW)
    v_max_absoluta = 3.0;      % [m/s] Límite mecánico de velocidad
    a_max_limite = 0.75;       % [m/s^2] Límite de aceleración de izaje
    
    % 1. CALCULO DE VELOCIDAD MAXIMA POR POTENCIA CONSTANTE (Hipérbola)
    % v_max = P / (m * g)
    v_potencia = P_const / (masa_total * g);
    
    % La velocidad límite es el menor valor entre la capacidad del motor y el límite mecánico
    v_max_limite = min(v_max_absoluta, v_potencia);
    
    % 2. ESCUDO DE ESPERA
    if t < t_inicio
        l_h_star = l_inicial;
        dl_h_star = 0;
        ddl_h_star = 0;
        return;
    end
    
    % Reloj interno de la maniobra
    t_eff = t - t_inicio;
    
    % Distancia a recorrer (longitud de cable a enrollar/desenrollar)
    D = abs(l_final - l_inicial);
    dir = sign(l_final - l_inicial); % +1 baja la carga, -1 sube la carga
    
    if D == 0
        l_h_star = l_inicial;
        dl_h_star = 0;
        ddl_h_star = 0;
        return;
    end
    
    % ---------------------------------------------------------------------
    % CALCULO DEL PERFIL CINEMATICO
    % ---------------------------------------------------------------------
    t_a = v_max_limite / a_max_limite;
    d_a = 0.5 * a_max_limite * t_a^2;
    
    if 2 * d_a >= D
        % Perfil Triangular (Tramos muy cortos)
        v_pico = sqrt(D * a_max_limite);
        t_a = v_pico / a_max_limite;
        t_crucero = 0;
        v_crucero = v_pico;
        d_crucero = 0;
        d_a = 0.5 * a_max_limite * t_a^2;
    else
        % Perfil Trapezoidal clásico
        v_crucero = v_max_limite;
        d_crucero = D - 2 * d_a;
        t_crucero = d_crucero / v_crucero;
    end
    
    t_total = 2 * t_a + t_crucero;
    
    % ---------------------------------------------------------------------
    % EVALUACION INSTANTANEA
    % ---------------------------------------------------------------------
    if t_eff < t_a
        % Fase 1: Aceleración
        ddl_h_star = a_max_limite * dir;
        dl_h_star = a_max_limite * t_eff * dir;
        l_h_star = l_inicial + 0.5 * a_max_limite * t_eff^2 * dir;
        
    elseif t_eff < (t_a + t_crucero)
        % Fase 2: Velocidad Constante (Crucero)
        t_fase2 = t_eff - t_a;
        ddl_h_star = 0;
        dl_h_star = v_crucero * dir;
        l_h_star = l_inicial + d_a * dir + v_crucero * t_fase2 * dir;
        
    elseif t_eff < t_total
        % Fase 3: Desaceleración
        t_fase3 = t_eff - (t_a + t_crucero);
        ddl_h_star = -a_max_limite * dir;
        dl_h_star = (v_crucero - a_max_limite * t_fase3) * dir;
        l_h_star = l_inicial + (d_a + d_crucero) * dir + (v_crucero * t_fase3 - 0.5 * a_max_limite * t_fase3^2) * dir;
        
    else
        % Fase 4: Posición final
        l_h_star = l_final;
        dl_h_star = 0;
        ddl_h_star = 0;
    end
end
